simulink model "c2_1chuanlianshixian"  (R2019b)
settings: Solver=VariableStepAuto  StartTime=0.0  StopTime=80  RelTol=1e-3
settings Model: Creator=wy151  LastModifiedBy=wy151

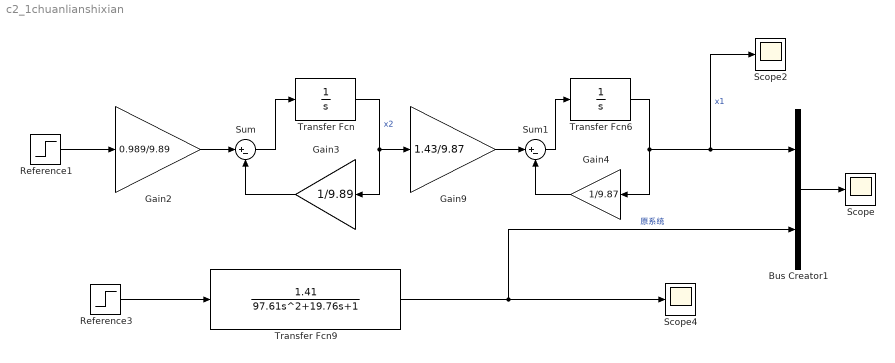
== system c2_1chuanlianshixian ==
  Bus Creator1 : BusCreator  Inputs=2
  Gain2 : Gain  Gain=0.989/9.89
  Gain3 : Gain  Gain=1/9.89
  Gain4 : Gain  Gain=1/9.87
  Gain9 : Gain  Gain=1.43/9.87
  Reference1 : Step  SampleTime=0
  Reference3 : Step  SampleTime=0
  Scope : Scope
  Scope2 : Scope
  Scope4 : Scope
  Sum : Sum  Inputs=|+-
  Sum1 : Sum  Inputs=|+-
  Transfer Fcn : TransferFcn  Denominator=[1 0]
  Transfer Fcn6 : TransferFcn  Denominator=[1 0]
  Transfer Fcn9 : TransferFcn  Numerator=[1.41]  Denominator=[97.61 19.76 1]
  wires:
  Reference3/1 -> Transfer Fcn9/1
  Sum/1 -> Transfer Fcn/1
  Reference1/1 -> Gain2/1
  Bus Creator1/1 -> Scope/1
  Transfer Fcn9/1 -> Scope4/1, Bus Creator1/2  "原系统"
  Gain9/1 -> Sum1/1
  Gain3/1 -> Sum/2
  Sum1/1 -> Transfer Fcn6/1
  Transfer Fcn6/1 -> Gain4/1, Scope2/1, Bus Creator1/1  "x1"
  Gain4/1 -> Sum1/2
  Transfer Fcn/1 -> Gain3/1, Gain9/1  "x2"
  Gain2/1 -> Sum/1
